simulink model "test_07"  (R2022b)
settings: Solver=FixedStepAuto  StartTime=0.0  StopTime=50  FixedStep=0.01  RelTol=1e-3  EnableMultiTasking=on
libraries: arduinolib x2, arduinosensorlib x1, simulink_extras x1
settings Model: ExtModeTrigDuration=2  Creator=laksh  LastModifiedBy=laksh
settings SolverCC: AutoInsertRateTranBlk=on
settings OptimizationCC: EnhancedBackFolding=on  PassReuseOutputArgsAs=Individual arguments  ZeroExternalMemoryAtStartup=off  ZeroInternalMemoryAtStartup=off  MaxStackSize=64  OptimizeBlockOrder=speed  DifferentSizesBufferReuse=on  OptimizationCustomize=off  EfficientTunableParamExpr=on
settings DebuggingCC: ParameterTunabilityLossMsg=error
settings HardwareCC: ProdBitPerInt=16  ProdBitPerPointer=16  ProdBitPerSizeT=16  ProdBitPerPtrDiffT=16  ProdLargestAtomicFloat=None  ProdWordSize=8  ProdHWDeviceType=Atmel->AVR
settings SFSimCC: MATLABDynamicMemAlloc=off
settings RTWCC: Description=Embedded Coder  SystemTargetFile=ert.tlc  HardwareBoard=Arduino Mega 2560  TLCOptions=-aInlineSetEventsForThisBaseRateFcn=TLC_FALSE -aSuppressMultiTaskScheduler=TLC_FALSE -aRateBasedStepFcn=1  TemplateMakefile=ert_default_tmf  Toolchain=Arduino AVR  BuildConfiguration=Faster Runs
settings CodeAppCC: ForceParamTrailComments=on  IgnoreCustomStorageClasses=off  OperatorAnnotations=on  SimulinkDataObjDesc=on  SFDataObjDesc=on  InsertBlockDesc=on
settings ERTTargetCC: SupportContinuousTime=on  SupportVariableSizeSignals=on  ExtModeTransport=3  ExtModeStaticAlloc=on  ExtModeAutomaticAllocSize=off  ExtModeStaticAllocSize=2048  ExtModeMexFile=ext_xcp  ExtModeIntrfLevel=Level2 - Open

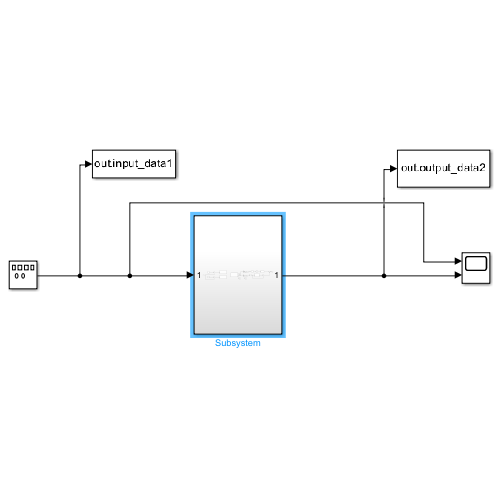
[thumbnail: Simulink's stored preview of the top-level diagram]
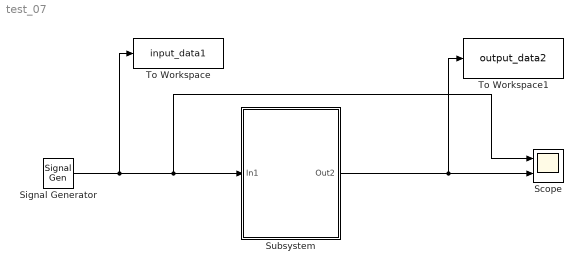
== system test_07 ==
  Scope : Scope  NumInputPorts=2
  Signal Generator : SignalGenerator  WaveForm=square  Frequency=1/20
  Subsystem : Subsystem
  To Workspace : ToWorkspace  VariableName=input_data1  SampleTime=-1
  To Workspace1 : ToWorkspace  VariableName=output_data2  SampleTime=-1
  wires:
  Signal Generator/1 -> To Workspace/1, Scope/1, Subsystem/1(In1)
  Subsystem/1(Out2) -> To Workspace1/1, Scope/2

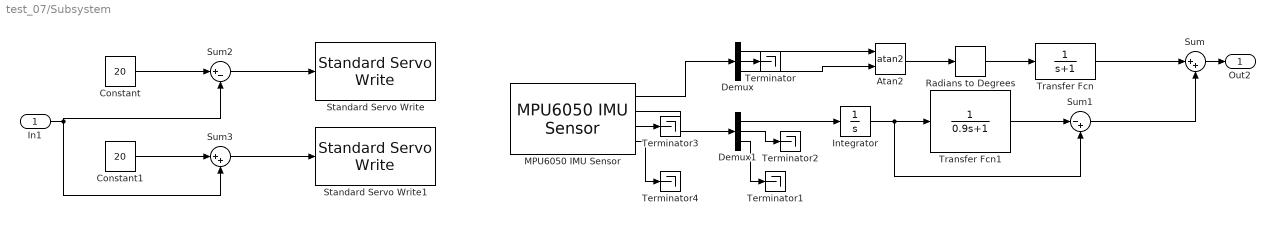
== system test_07/Subsystem ==
  In1 : Inport
  Atan2 : Trigonometry  Operator=atan2
  Constant : Constant  Value=20
  Constant1 : Constant  Value=20
  Demux : Demux  Outputs=3
  Demux1 : Demux  Outputs=3
  Integrator : Integrator
  MPU6050 IMU Sensor : arduinosensorlib/MPU6050 IMU Sensor  SlaveAddress=0x68  Accel=on  AngularRate=on  Temperature=on  Status=on  Timestamp=off  EulerAngles=off  Quat=off  AccelRange=2G  GyroRange=250 dps  DmpOdr=200 Hz  Dlpf=Accelerometer: 184Hz, Gyroscope: 188Hz  spf=1  SampleTime=-1  QueueSizeFactor=1
  Radians to Degrees : simulink_extras/Transformations/Radians to Degrees
  Standard Servo Write : arduinolib/Standard Servo Write  pinNumber=3  ServoIndex=0  blockPlatform=ARDUINO
  Standard Servo Write1 : arduinolib/Standard Servo Write  pinNumber=5  ServoIndex=1  blockPlatform=ARDUINO
  Sum : Sum  Inputs=|++
  Sum1 : Sum  Inputs=|-+
  Sum2 : Sum  Inputs=|+-
  Sum3 : Sum  Inputs=|++
  Terminator{,1..4} (5 alike) : Terminator
  Transfer Fcn : TransferFcn  Denominator=[1 1]
  Transfer Fcn1 : TransferFcn  Denominator=[0.9 1]
  Out2 : Outport
  wires:
  Sum1/1 -> Sum/2
  Constant1/1 -> Sum3/1
  Transfer Fcn1/1 -> Sum1/1
  Demux1/1 -> Integrator/1
  MPU6050 IMU Sensor/1 -> Demux/1
  Transfer Fcn/1 -> Sum/1
  MPU6050 IMU Sensor/2 -> Demux1/1
  Atan2/1 -> Radians to Degrees/1
  Sum3/1 -> Standard Servo Write1/1
  Radians to Degrees/1 -> Transfer Fcn/1
  Demux/1 -> Atan2/1
  Sum/1 -> Out2/1
  Constant/1 -> Sum2/1
  Demux/3 -> Atan2/2
  Integrator/1 -> Sum1/2, Transfer Fcn1/1
  In1/1 -> Sum2/2, Sum3/2
  Sum2/1 -> Standard Servo Write/1
  MPU6050 IMU Sensor/3 -> Terminator3/1
  Demux/2 -> Terminator/1
  Demux1/3 -> Terminator1/1
  Demux1/2 -> Terminator2/1
  MPU6050 IMU Sensor/4 -> Terminator4/1
